simulink model "ground_sim"  (R2022a)
settings: Solver=FixedStepAuto  StartTime=0.0  StopTime=35  FixedStep=framePeriod_s  RelTol=1e-9
values from neighbouring files (symbols this model uses):
  framePeriod_s = 1/frameRate_hz    (= 0.02)    [autocode_setup.m]    (also in setup.m)
undefined symbols (not defined in the file or in its folder): accel_mps2, Aircraft, alt_msl_m, alt_wgs84_m, datetime, datevec, die_temp_c, Earth, Env, Fmu, gyro_radps, hdop, healthy, horz_acc_m, imu_healthy, InitCond, lat_rad, lon_rad, mag_healthy, mag_ut, ned_vel_mps, new_data, new_imu_data, new_mag_data, num_sats, pres_pa, spd_mps, Telem, tow_ms, track_acc_rad, track_rad, vdop, vel_acc_mps, vert_acc_m, week, WGS84
libraries: simulink x8, aerolibconvert2 x5, aerolibasang x3, aerolibtransform2 x2, aerolibgravity2 x2, aerolibatmos2 x1, sharedtransform x1, uavutilslib x1
(part 1 of 4)
settings Model: Creator=brian  LastModifiedBy=remoteuser
settings SolverCC: AlgebraicLoopSolver=TrustRegion
settings DataIOCC: SaveOutput=off  SignalLogging=off  DSMLogging=off  SaveTime=off  ReturnWorkspaceOutputsName=Data
settings OptimizationCC: DefaultParameterBehavior=Inlined  EnhancedBackFolding=on  PassReuseOutputArgsAs=Individual arguments  ZeroExternalMemoryAtStartup=off  ZeroInternalMemoryAtStartup=off  OptimizeBlockOrder=speed  DifferentSizesBufferReuse=on  OptimizationCustomize=off  EfficientTunableParamExpr=on
settings DebuggingCC: Int32ToFloatConvMsg=none  ParameterPrecisionLossMsg=none  ParameterTunabilityLossMsg=error  UnconnectedInputMsg=warning  UnconnectedOutputMsg=warning  UnconnectedLineMsg=warning  SFMachineParentedDataDiag=warning
settings SFSimCC: MATLABDynamicMemAlloc=off
settings RTWCC: SystemTargetFile=ert.tlc  GenCodeOnly=on  TemplateMakefile=ert_default_tmf  DLArmComputeVersion=19.05
settings CodeAppCC: ForceParamTrailComments=on  IgnoreCustomStorageClasses=off  OperatorAnnotations=on  SimulinkDataObjDesc=on  SFDataObjDesc=on  InsertBlockDesc=on
settings ERTTargetCC: TargetLangStandard=C99 (ISO)  GenerateSampleERTMain=on  InlinedParameterPlacement=NonHierarchical  ERTCustomFileTemplate=example_file_process.tlc

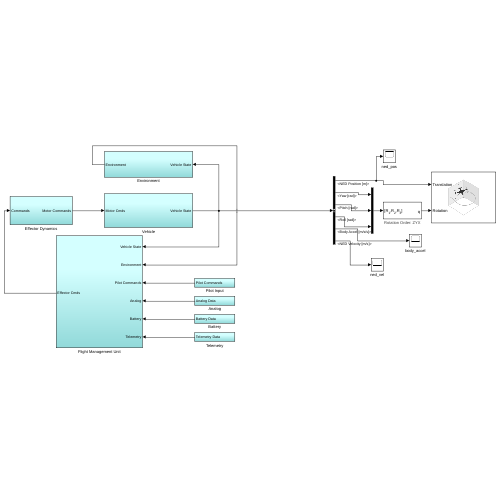
[thumbnail: Simulink's stored preview of the top-level diagram]
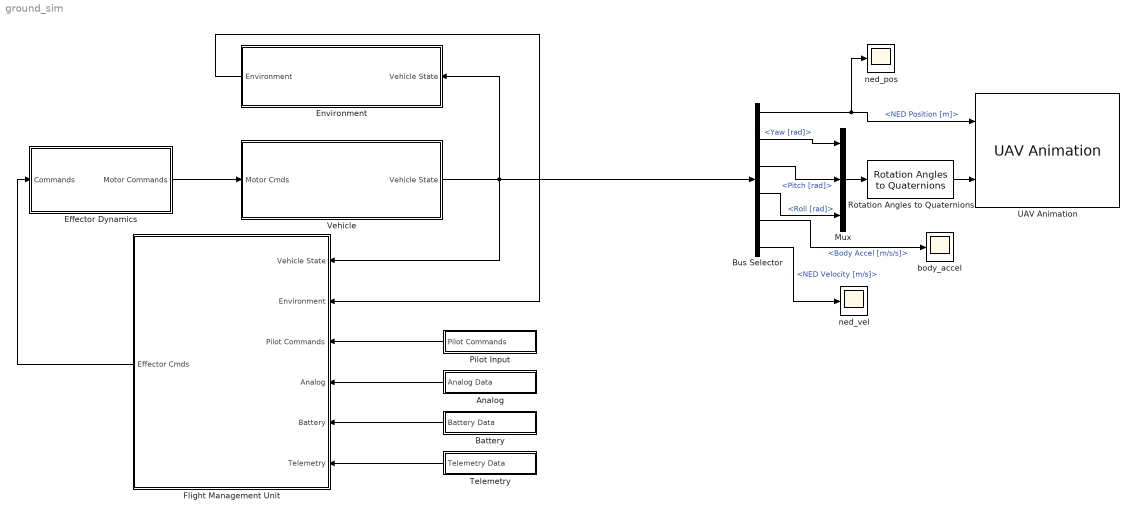
== system ground_sim ==
  Analog : Subsystem
  Battery : Subsystem
  Bus Selector : BusSelector  OutputSignals=NED Position [m],Yaw [rad],Pitch [rad],Roll [rad],Body Accel [m/s/s],NED Velocity [m/s]
  Effector Dynamics : Subsystem
  Environment : Subsystem
  Flight Management Unit : Subsystem
  Mux : Mux  Inputs=3
  Pilot Input : Subsystem
  Rotation Angles to Quaternions : sharedtransform/Rotation Angles to Quaternions  rotationOrder=ZYX  aMode=aMode
      settings: SourceProductBaseCode=AE,PW,DR,MT,VE
  Telemetry : Subsystem
  UAV Animation : uavutilslib/UAV Animation  UAVType=Multirotor  UAVSize=1  InertialZDirection=Down  SampleTime=-1
      settings: SourceProductBaseCode=UV
  Vehicle : Subsystem
  body_accel : Scope
  ned_pos : Scope
  ned_vel : Scope
  wires:
  Pilot Input/1(Pilot Commands) -> Flight Management Unit/3(Pilot Commands)
  Environment/1(Environment) -> Flight Management Unit/2(Environment)
  Effector Dynamics/1(Motor Commands) -> Vehicle/1(Motor Cmds)
  Telemetry/1(Telemetry Data) -> Flight Management Unit/6(Telemetry)
  Flight Management Unit/1(Effector Cmds) -> Effector Dynamics/1(Commands)
  Analog/1(Analog Data) -> Flight Management Unit/4(Analog)
  Battery/1(Battery Data) -> Flight Management Unit/5(Battery)
  Bus Selector/6 -> ned_vel/1  "<NED Velocity [m/s]>"
  Bus Selector/2 -> Mux/1  "<Yaw [rad]>"
  Bus Selector/5 -> body_accel/1  "<Body Accel [m/s/s]>"
  Rotation Angles to Quaternions/1 -> UAV Animation/2
  Bus Selector/3 -> Mux/2  "<Pitch [rad]>"
  Bus Selector/4 -> Mux/3  "<Roll [rad]>"
  Mux/1 -> Rotation Angles to Quaternions/1
  Bus Selector/1 -> ned_pos/1, UAV Animation/1  "<NED Position [m]>"
  Vehicle/1(Vehicle State) -> Bus Selector/1, Environment/1(Vehicle State), Flight Management Unit/1(Vehicle State)

== system ground_sim/Analog ==
  note: Raw voltages measured at the FMU, should be between
      | 0 and 3.3V
  Bus Creator : BusCreator  Inputs=1
  Constant : Constant  Value=zeros(1, Fmu.NUM_AIN)
  Mux : Mux  Inputs=2
  Random Number : RandomNumber  Mean=0.8  Variance=0.01  SampleTime=framePeriod_s
  Selector1 : Selector  InputPortWidth=Fmu.NUM_AIN  IndexOptions=Starting index (dialog)  Indices=[2]  OutputSizes=Fmu.NUM_AIN-1
  Analog Data : Outport
  wires:
  Bus Creator/1 -> Analog Data/1
  Mux/1 -> Bus Creator/1  "Voltages"
  Random Number/1 -> Mux/1
  Selector1/1 -> Mux/2
  Constant/1 -> Selector1/1  "Voltages"

== system ground_sim/Battery ==
  note: This is the amp draw from the battery
  note: The mRo Power Zero module
      | outputs 1V for 33.594 amps drawn
      | from the battery
  note: This is the voltage measured by the FMU
      | power port. It is typically the current, scaled
      | by the power module mA / volt
  note: This is the voltage
      | measured by the FMU at
      | the power port. It is typically
      | the battery voltage scaled by the
      | power module voltage divider.
  note: The mRo Power Zero module
      | outputs 1V for 15.30 V at the
      | battery
  Bus Creator : BusCreator  Inputs=2
  Constant : Constant  Value=Aircraft.Battery.voltage
  Constant1 : Constant  Value=42
  Constant2 : Constant
  Constant3 : Constant
  Divide : Product  Inputs=*/
  Divide1 : Product  Inputs=*/
  Battery Data : Outport
  wires:
  Bus Creator/1 -> Battery Data/1
  Constant2/1 -> Divide/2
  Constant1/1 -> Divide/1
  Divide/1 -> Bus Creator/2  "Current [V]"
  Divide1/1 -> Bus Creator/1  "Voltage [V]"
  Constant/1 -> Divide1/1
  Constant3/1 -> Divide1/2

== system ground_sim/Effector Dynamics ==
  Commands : Inport
  Bus Selector : BusSelector  OutputSignals=PWM.Cmds
  Selector1 : Selector  InputPortWidth=Aircraft.Eff.nPwm  IndexOptions=Index vector (dialog)  Indices=Aircraft.Motor.map  OutputSizes=1
  Motor Commands : Outport
  wires:
  Bus Selector/1 -> Selector1/1  "<Cmds>"
  Commands/1 -> Bus Selector/1
  Selector1/1 -> Motor Commands/1

== system ground_sim/Environment ==
  note: nT to uT conversion
  Vehicle State : Inport
  Angle Conversion4 : aerolibconvert2/Angle Conversion  IU=rad  OU=deg
  Angle Conversion5 : aerolibconvert2/Angle Conversion  IU=rad  OU=deg
  Bus Creator : BusCreator  Inputs=6
  Bus Selector : BusSelector  OutputSignals=Latitude [rad],Longitude [rad],Altitude WGS84 [m],Altitude MSL [m]
  COESA Atmosphere Model : aerolibatmos2/COESA Atmosphere Model  units=Metric (MKS)  spec=1976 COESA-extended U.S. Standard Atmosphere  model=Profile  profile_var=High temperature  profile_percent=1%  profile_alt=5 km (16404 ft)  envelope_var=High temperature  envelope_percent=1%  action=Warning
  Constant : Constant  Value=Env.wmm_nt
  Gain : Gain  Gain=1e-3
  Mux : Mux  Inputs=3
  "WGS84 Gravity Model  " : GravityWGS84
  Environment : Outport
  wires:
  [lon_deg] -> Mux/2
  COESA Atmosphere Model/4 -> Bus Creator/4  "Density [kg/m^3]"
  Mux/1 -> "WGS84 Gravity Model  "/1
  Bus Selector/3 -> [alt_wgs84_m]  "<Altitude WGS84 [m]>"
  Vehicle State/1 -> Bus Selector/1
  Bus Selector/2 -> Angle Conversion5/1  "<Longitude [rad]>"
  COESA Atmosphere Model/2 -> Bus Creator/2  "Speed of Sound [m/s]"
  Bus Selector/4 -> COESA Atmosphere Model/1  "<Altitude MSL [m]>"
  [alt_wgs84_m] -> Mux/3
  Angle Conversion4/1 -> [lat_deg]
  [lat_deg] -> Mux/1
  Bus Creator/1 -> Environment/1
  Constant/1 -> Gain/1
  Gain/1 -> Bus Creator/6  "Magnetic Field [uT]"
  "WGS84 Gravity Model  "/1 -> Bus Creator/5  "Gravity [m/s/s]"
  Bus Selector/1 -> Angle Conversion4/1  "<Latitude [rad]>"
  COESA Atmosphere Model/3 -> Bus Creator/3  "Pressure [Pa]"
  COESA Atmosphere Model/1 -> Bus Creator/1  "Temperature [K]"
  Angle Conversion5/1 -> [lon_deg]

== system ground_sim/Flight Management Unit ==
  Vehicle State : Inport
  Environment : Inport  Port=2
  Pilot Commands : Inport  Port=3
  Analog : Inport  Port=4
  Battery : Inport  Port=5
  Telemetry : Inport  Port=6
  Bus Selector1 : BusSelector  OutputSignals=Waypoint Reached
  Bus Selector2 : BusSelector  OutputSignals=Waypoint Reached,SBUS,PWM  OutputAsBus=on
  Navigation Filter Model : Subsystem
      settings: PortSchema="{\"entries\":[{\"content\":{\"sides\":[{\"content\":{\"connectorIds\":[]},\"type\":\"ConnectorPlacement.EquallySpacedRectSide\",\"uuid\":\"b20f7590-d69b-48b8-beb1-2fb7d3ab0357\"},{\"content\":{\"connectorIds\":[],\"side\":\"RIGHT\"},\"type\":\"ConnectorPlacement.EquallySpacedRectSide\",\"uuid\":\"07801f8a-7756-483e-a050-3c2fccc33404\"},{\"content\":{\"connectorIds\":[\"In1\",\"In2\"],\"side\":\"TOP\"},\"type\":\"ConnectorPlacement.EquallySpacedRectSide\",\"uuid\":\"ce3c3c94-ed36-4103-b079-69dcaeaf21e9\"},{\"content\":{\"connectorIds\":[\"Out1\"],\"side\":\"BOTTOM\"},\"type\":\"ConnectorPlacement.EquallySpacedRectSide\",\"uuid\":\"ba78b819-a471-4bc3-b479-e6a973cfe14f\"},{\"content\":{\"connectorIds\":[],\"side\":\"HIDDEN\"},\"type\":\"ConnectorPlacement.EquallySpacedRectSide\",\"uuid\":\"3cf915a5-25a1-4380-9090-9561533312da\"}]},\"type\":\"ConnectorPlacement.EquallySpacedConnector\",\"uuid\":\"7ef4ddaa-ccd2-4778-89ce-8b4685524e82\"}],\"packageUris\":[\"http://schema.mathworks.com/mf0/Connector/R2020b\"],\"version\":\"1.0\"}"
  Sensor Models : Subsystem
      settings: PortSchema="{\"entries\":[{\"content\":{\"sides\":[{\"content\":{\"connectorIds\":[]},\"type\":\"ConnectorPlacement.EquallySpacedRectSide\",\"uuid\":\"b20f7590-d69b-48b8-beb1-2fb7d3ab0357\"},{\"content\":{\"connectorIds\":[],\"side\":\"RIGHT\"},\"type\":\"ConnectorPlacement.EquallySpacedRectSide\",\"uuid\":\"07801f8a-7756-483e-a050-3c2fccc33404\"},{\"content\":{\"connectorIds\":[\"In1\",\"In2\",\"In3\",\"In4\",\"In5\"],\"side\":\"TOP\"},\"type\":\"ConnectorPlacement.EquallySpacedRectSide\",\"uuid\":\"ce3c3c94-ed36-4103-b079-69dcaeaf21e9\"},{\"content\":{\"connectorIds\":[\"Out1\"],\"side\":\"BOTTOM\"},\"type\":\"ConnectorPlacement.EquallySpacedRectSide\",\"uuid\":\"ba78b819-a471-4bc3-b479-e6a973cfe14f\"},{\"content\":{\"connectorIds\":[],\"side\":\"HIDDEN\"},\"type\":\"ConnectorPlacement.EquallySpacedRectSide\",\"uuid\":\"3cf915a5-25a1-4380-9090-9561533312da\"}]},\"type\":\"ConnectorPlacement.EquallySpacedConnector\",\"uuid\":\"7ef4ddaa-ccd2-4778-89ce-8b4685524e82\"}],\"packageUris\":[\"http://schema.mathworks.com/mf0/Connector/R2020b\"],\"version\":\"1.0\"}"
  Subsystem : Subsystem
  System Model : Subsystem
      settings: PortSchema="{\"entries\":[{\"content\":{\"sides\":[{\"content\":{\"connectorIds\":[]},\"type\":\"ConnectorPlacement.EquallySpacedRectSide\",\"uuid\":\"b20f7590-d69b-48b8-beb1-2fb7d3ab0357\"},{\"content\":{\"connectorIds\":[],\"side\":\"RIGHT\"},\"type\":\"ConnectorPlacement.EquallySpacedRectSide\",\"uuid\":\"07801f8a-7756-483e-a050-3c2fccc33404\"},{\"content\":{\"connectorIds\":[],\"side\":\"TOP\"},\"type\":\"ConnectorPlacement.EquallySpacedRectSide\",\"uuid\":\"ce3c3c94-ed36-4103-b079-69dcaeaf21e9\"},{\"content\":{\"connectorIds\":[\"Out1\"],\"side\":\"BOTTOM\"},\"type\":\"ConnectorPlacement.EquallySpacedRectSide\",\"uuid\":\"ba78b819-a471-4bc3-b479-e6a973cfe14f\"},{\"content\":{\"connectorIds\":[],\"side\":\"HIDDEN\"},\"type\":\"ConnectorPlacement.EquallySpacedRectSide\",\"uuid\":\"3cf915a5-25a1-4380-9090-9561533312da\"}]},\"type\":\"ConnectorPlacement.EquallySpacedConnector\",\"uuid\":\"7ef4ddaa-ccd2-4778-89ce-8b4685524e82\"}],\"packageUris\":[\"http://schema.mathworks.com/mf0/Connector/R2020b\"],\"version\":\"1.0\"}"
  Unit Delay : UnitDelay  SampleTime=-1  HasFrameUpgradeWarning=on
  Unit Delay1 : UnitDelay  SampleTime=-1  HasFrameUpgradeWarning=on
  Vehicle Management System (VMS) : Subsystem  TreatAsAtomicUnit=on
  Effector Cmds : Outport
  wires:
  Environment/1 -> Navigation Filter Model/1(Environment), Sensor Models/1(Environment)
  Vehicle State/1 -> Navigation Filter Model/2(Vehicle State), Sensor Models/2(Vehicle State)
  Sensor Models/1(Sensors) -> Unit Delay/1
  Navigation Filter Model/1(Navigation Filter Data) -> Unit Delay1/1
  System Model/1(System) -> Vehicle Management System (VMS)/1(System Data)
  Pilot Commands/1 -> Sensor Models/3(Inceptor Data)
  Telemetry/1 -> Subsystem/1(Bus)
  Vehicle Management System (VMS)/1(VMS Data) -> Bus Selector2/1
  Unit Delay/1 -> Vehicle Management System (VMS)/2(Sensor Data)
  Unit Delay1/1 -> Vehicle Management System (VMS)/3(Navigation Filter Data)
  Analog/1 -> Sensor Models/4(Analog Data)
  Battery/1 -> Sensor Models/5(Battery Data)
  Subsystem/1(Telemetry Data) -> Vehicle Management System (VMS)/4(Telemetry Data)
  Bus Selector1/1 -> Subsystem/2(<Waypoint Reached>)  "<Waypoint Reached>"
  Bus Selector2/1 -> Bus Selector1/1, Effector Cmds/1

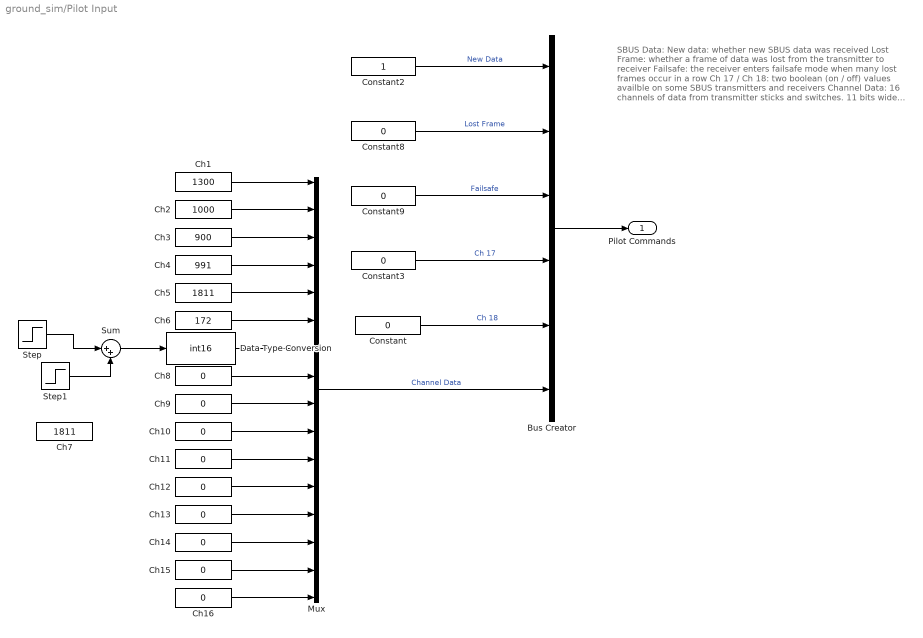
== system ground_sim/Pilot Input ==
  note: SBUS Data:
      | New data: whether new SBUS data was received
      | Lost Frame: whether a frame of data was lost from the transmitter to receiver
      | Failsafe: the receiver enters failsafe mode when many lost frames occur in a row
      | Ch 17 / Ch 18: two boolean (on / off) values availble on some SBUS transmitters and receivers
      | Channel Data: 16 channels of data from transmitter sticks and switches. 11 bits wide limiting values to 0 - 2048. Actual ranges may be different, for example, FrSky typically uses 172 - 1811 unless its range is extended to +/- 150%
  Bus Creator : BusCreator  Inputs=6
  Ch1 : Constant  Value=1300  OutDataTypeStr=int16  SampleTime=-1
  Ch{8..16} (9 alike) : Constant  Value=0  OutDataTypeStr=int16  SampleTime=-1
  Ch2 : Constant  Value=1000  OutDataTypeStr=int16  SampleTime=-1
  Ch3 : Constant  Value=900  OutDataTypeStr=int16  SampleTime=-1
  Ch4 : Constant  Value=991  OutDataTypeStr=int16  SampleTime=-1
  Ch5 : Constant  Value=1811  OutDataTypeStr=int16  SampleTime=-1
  Ch6 : Constant  Value=172  OutDataTypeStr=int16  SampleTime=-1
  Ch7 : Constant  Value=1811  OutDataTypeStr=int16  SampleTime=-1
  Constant : Constant  Value=0  OutDataTypeStr=int8
  Constant2 : Constant  OutDataTypeStr=boolean
  Constant3 : Constant  Value=0  OutDataTypeStr=boolean
  Constant8 : Constant  Value=0  OutDataTypeStr=boolean
  Constant9 : Constant  Value=0  OutDataTypeStr=boolean
  Data Type Conversion : DataTypeConversion  OutDataTypeStr=int16  SaturateOnIntegerOverflow=off  RndMeth=Floor
  Mux : Mux  Inputs=16
  Step : Step  Time=0  After=1811  SampleTime=0
  Step1 : Step  Time=2*framePeriod_s  After=-1811  SampleTime=0
  Sum : Sum  Inputs=|++
  Pilot Commands : Outport
  wires:
  Bus Creator/1 -> Pilot Commands/1
  Constant2/1 -> Bus Creator/1  "New Data"
  Constant8/1 -> Bus Creator/2  "Lost Frame"
  Constant9/1 -> Bus Creator/3  "Failsafe"
  Constant3/1 -> Bus Creator/4  "Ch 17"
  Constant/1 -> Bus Creator/5  "Ch 18"
  Mux/1 -> Bus Creator/6  "Channel Data"
  Ch1/1 -> Mux/1
  Ch16/1 -> Mux/16
  Ch15/1 -> Mux/15
  Ch14/1 -> Mux/14
  Ch13/1 -> Mux/13
  Ch12/1 -> Mux/12
  Ch11/1 -> Mux/11
  Ch10/1 -> Mux/10
  Ch9/1 -> Mux/9
  Ch8/1 -> Mux/8
  Data Type Conversion/1 -> Mux/7
  Ch6/1 -> Mux/6
  Ch4/1 -> Mux/4
  Ch2/1 -> Mux/2
  Ch3/1 -> Mux/3
  Ch5/1 -> Mux/5
  Step/1 -> Sum/1
  Step1/1 -> Sum/2
  Sum/1 -> Data Type Conversion/1

== system ground_sim/Telemetry ==
  Bus Creator : BusCreator  Inputs=11
  Constant1 : Constant  Value=0  OutDataTypeStr=boolean
  Constant10 : Constant  Value=Telem.Fence  OutDataTypeStr=Bus: MissionItem
  Constant11 : Constant  Value=Telem.Rally  OutDataTypeStr=Bus: MissionItem
  Constant2 : Constant  Value=0  OutDataTypeStr=boolean
  Constant3 : Constant  OutDataTypeStr=int16
  Constant4 : Constant  Value=0  OutDataTypeStr=int16
  Constant5 : Constant  Value=0  OutDataTypeStr=int16
  Constant6 : Constant  Value=0  OutDataTypeStr=int16
  Constant7 : Constant  Value=[0 0 0 0 0 0 0 0 0 0 1 1 1 0 0 0 0 0 0 0 0 0 0 0]  OutDataTypeStr=boolean
  Constant8 : Constant  Value=0  OutDataTypeStr=boolean
  Constant9 : Constant  Value=Telem.FlightPlan  OutDataTypeStr=Bus: MissionItem
  Telemetry Data : Outport
  wires:
  Bus Creator/1 -> Telemetry Data/1
  Constant8/1 -> Bus Creator/1  "Waypoints Updated"
  Constant1/1 -> Bus Creator/2  "Fence Updated"
  Constant2/1 -> Bus Creator/3  "Rally Points Updated"
  Constant3/1 -> Bus Creator/4  "Current Waypoint Index"
  Constant4/1 -> Bus Creator/5  "Number of Waypoints"
  Constant5/1 -> Bus Creator/6  "Number of Fence Points"
  Constant6/1 -> Bus Creator/7  "Number of Rally Points"
  Constant7/1 -> Bus Creator/8  "Parameters"
  Constant9/1 -> Bus Creator/9  "Flight Plan"
  Constant10/1 -> Bus Creator/10  "Fence"
  Constant11/1 -> Bus Creator/11  "Rally"

== system ground_sim/Vehicle ==
  note: The dynamics can be input here using the Motor Cmds as input
  Motor Cmds : Inport
  Bus Creator : BusCreator  Inputs=26
  Demux : Demux  Outputs=3
  Ground : Ground
  MATLAB Function : MATLAB Function  TreatAsAtomicUnit=on
  Vehicle Model : Subsystem
  Vehicle State : Outport
  wires:
  Vehicle Model/20(Angle of Attack Rate [rad/s]) -> Bus Creator/20  "Angle of Attack Rate [rad/s]"
  Vehicle Model/4(Altitude MSL [m]) -> Bus Creator/4  "Altitude MSL [m]"
  Vehicle Model/26(DCM_be) -> Bus Creator/26  "DCM_be"
  Vehicle Model/16(Dynamic Pressure [Pa]) -> Bus Creator/16  "Dynamic Pressure [Pa]"
  Vehicle Model/22(Sideslip Angle Rate [rad/s]) -> Bus Creator/22  "Sideslip Angle Rate [rad/s]"
  Vehicle Model/21(Sideslip Angle [rad]) -> Bus Creator/21  "Sideslip Angle [rad]"
  Vehicle Model/24(Flight Path Angle [rad]) -> Bus Creator/24  "Flight Path Angle [rad]"
  Vehicle Model/11(Yaw [rad]) -> MATLAB Function/2(phi), Bus Creator/11  "Yaw [rad]"
  Vehicle Model/18(Mach) -> Bus Creator/18  "Mach"
  Vehicle Model/5(Altitude AGL [m]) -> Bus Creator/5  "Altitude AGL [m]"
  Vehicle Model/6(NED Position [m]) -> Bus Creator/6  "NED Position [m]"
  Vehicle Model/23(Ground Track [rad]) -> Bus Creator/23  "Ground Track [rad]"
  Vehicle Model/10(Roll [rad]) -> Bus Creator/10  "Roll [rad]"
  Vehicle Model/7(NED Velocity [m/s]) -> Bus Creator/7  "NED Velocity [m/s]"
  Vehicle Model/17(Airspeed [m/s]) -> Bus Creator/17  "Airspeed [m/s]"
  Vehicle Model/15(Body Rotational Accel [rad/s/s]) -> Bus Creator/15  "Body Rotational Accel [rad/s/s]"
  Vehicle Model/14(Body Rotational Rate [rad/s]) -> Bus Creator/14  "Body Rotational Rate [rad/s]"
  Vehicle Model/13(Body Accel [m/s/s]) -> Bus Creator/13  "Body Accel [m/s/s]"
  Vehicle Model/9(Pitch [rad]) -> Bus Creator/9  "Pitch [rad]"
  Vehicle Model/8(NED Accel [m/s/s]) -> Bus Creator/8  "NED Accel [m/s/s]"
  Bus Creator/1 -> Vehicle State/1
  Vehicle Model/19(Angle of Attack [rad]) -> Bus Creator/19  "Angle of Attack [rad]"
  Vehicle Model/3(Altitude WGS84 [m]) -> Bus Creator/3  "Altitude WGS84 [m]"
  Motor Cmds/1 -> MATLAB Function/1(u)
  Vehicle Model/2(Longitude [rad]) -> Bus Creator/2  "Longitude [rad]"
  Vehicle Model/1(Latitude [rad]) -> Bus Creator/1  "Latitude [rad]"
  Vehicle Model/12(Body Velocity [m/s]) -> Bus Creator/12  "Body Velocity [m/s]"
  Vehicle Model/25(Ground Speed [m/s]) -> Bus Creator/25  "Ground Speed [m/s]"
  Demux/1 -> Vehicle Model/1(v_x [mps])
  Demux/2 -> Vehicle Model/2(v_y [mps])
  Demux/3 -> Vehicle Model/3(phi_dot [radps])
  Ground/1 -> Vehicle Model/5(Speed of Sound [m/s]), Vehicle Model/4(Density [kg/m^3])
  MATLAB Function/1(rate_out) -> Demux/1

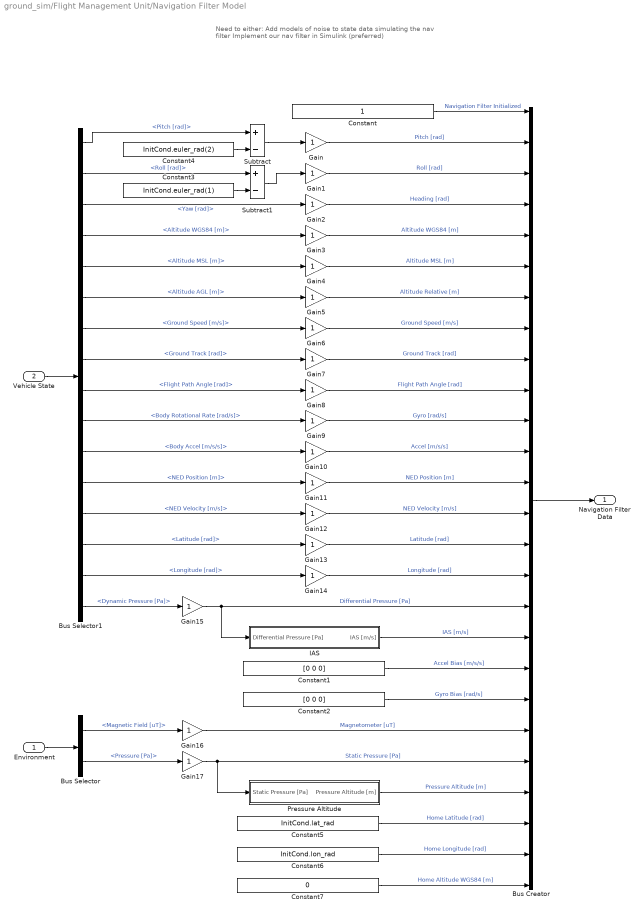
== system ground_sim/Flight Management Unit/Navigation Filter Model ==
  note: Need to either:
      | Add models of noise to state data simulating the nav filter
      | Implement our nav filter in Simulink (preferred)
  Environment : Inport
  Vehicle State : Inport  Port=2
  Bus Creator : BusCreator  Inputs=26
  Bus Selector : BusSelector  OutputSignals=Magnetic Field [uT],Pressure [Pa]
  Bus Selector1 : BusSelector  OutputSignals=Pitch [rad],Roll [rad],Yaw [rad],Altitude WGS84 [m],Altitude MSL [m],Altitude AGL [m],Ground Speed [m/s],Ground Track [rad],Flight Path Angle [rad],Body Rotational Rate [rad/s],Body Accel [m/s/s],NED Position [m],NED Velocity [m/s],Latitude [rad],Longitude [rad],Dynamic Pressure [Pa]
  Constant : Constant
  Constant1 : Constant  Value=[0 0 0]
  Constant2 : Constant  Value=[0 0 0]
  Constant3 : Constant  Value=InitCond.euler_rad(1)
  Constant4 : Constant  Value=InitCond.euler_rad(2)
  Constant5 : Constant  Value=InitCond.lat_rad
  Constant6 : Constant  Value=InitCond.lon_rad
  Constant7 : Constant  Value=0
  Gain{,1..17} (18 alike) : Gain
  IAS : Subsystem
  Pressure Altitude : Subsystem
  Subtract : Sum  Inputs=+-
  Subtract1 : Sum  Inputs=+-
  Navigation Filter Data : Outport
  wires:
  Environment/1 -> Bus Selector/1
  Bus Creator/1 -> Navigation Filter Data/1
  Vehicle State/1 -> Bus Selector1/1
  Constant/1 -> Bus Creator/1  "Navigation Filter Initialized"
  Bus Selector1/1 -> Subtract/1  "<Pitch [rad]>"
  Bus Selector1/2 -> Subtract1/1  "<Roll [rad]>"
  Bus Selector1/3 -> Gain2/1  "<Yaw [rad]>"
  Bus Selector1/4 -> Gain3/1  "<Altitude WGS84 [m]>"
  Bus Selector1/5 -> Gain4/1  "<Altitude MSL [m]>"
  Bus Selector1/6 -> Gain5/1  "<Altitude AGL [m]>"
  Bus Selector1/7 -> Gain6/1  "<Ground Speed [m/s]>"
  Bus Selector1/8 -> Gain7/1  "<Ground Track [rad]>"
  Bus Selector1/9 -> Gain8/1  "<Flight Path Angle [rad]>"
  Bus Selector1/10 -> Gain9/1  "<Body Rotational Rate [rad/s]>"
  Bus Selector1/11 -> Gain10/1  "<Body Accel [m/s/s]>"
  Bus Selector1/12 -> Gain11/1  "<NED Position [m]>"
  Bus Selector1/13 -> Gain12/1  "<NED Velocity [m/s]>"
  Bus Selector/2 -> Gain17/1  "<Pressure [Pa]>"
  Pressure Altitude/1(Pressure Altitude [m]) -> Bus Creator/23  "Pressure Altitude [m]"
  Bus Selector/1 -> Gain16/1  "<Magnetic Field [uT]>"
  Constant2/1 -> Bus Creator/20  "Gyro Bias [rad/s]"
  Constant1/1 -> Bus Creator/19  "Accel Bias [m/s/s]"
  IAS/1(IAS [m/s]) -> Bus Creator/18  "IAS [m/s]"
  Bus Selector1/16 -> Gain15/1  "<Dynamic Pressure [Pa]>"
  Bus Selector1/15 -> Gain14/1  "<Longitude [rad]>"
  Bus Selector1/14 -> Gain13/1  "<Latitude [rad]>"
  Gain/1 -> Bus Creator/2  "Pitch [rad]"
  Gain1/1 -> Bus Creator/3  "Roll [rad]"
  Gain2/1 -> Bus Creator/4  "Heading [rad]"
  Gain3/1 -> Bus Creator/5  "Altitude WGS84 [m]"
  Gain4/1 -> Bus Creator/6  "Altitude MSL [m]"
  Gain5/1 -> Bus Creator/7  "Altitude Relative [m]"
  Gain6/1 -> Bus Creator/8  "Ground Speed [m/s]"
  Gain7/1 -> Bus Creator/9  "Ground Track [rad]"
  Gain8/1 -> Bus Creator/10  "Flight Path Angle [rad]"
  Gain9/1 -> Bus Creator/11  "Gyro [rad/s]"
  Gain10/1 -> Bus Creator/12  "Accel [m/s/s]"
  Gain11/1 -> Bus Creator/13  "NED Position [m]"
  Gain12/1 -> Bus Creator/14  "NED Velocity [m/s]"
  Gain13/1 -> Bus Creator/15  "Latitude [rad]"
  Gain14/1 -> Bus Creator/16  "Longitude [rad]"
  Gain15/1 -> IAS/1(Differential Pressure [Pa]), Bus Creator/17  "Differential Pressure [Pa]"
  Gain16/1 -> Bus Creator/21  "Magnetometer [uT]"
  Gain17/1 -> Pressure Altitude/1(Static Pressure [Pa]), Bus Creator/22  "Static Pressure [Pa]"
  Subtract/1 -> Gain/1
  Subtract1/1 -> Gain1/1
  Constant3/1 -> Subtract1/2
  Constant4/1 -> Subtract/2
  Constant5/1 -> Bus Creator/24  "Home Latitude [rad]"
  Constant6/1 -> Bus Creator/25  "Home Longitude [rad]"
  Constant7/1 -> Bus Creator/26  "Home Altitude WGS84 [m]"

== system ground_sim/Flight Management Unit/Sensor Models ==
  Environment : Inport
  Vehicle State : Inport  Port=2
  Inceptor Data : Inport  Port=3
  Analog Data : Inport  Port=4
  Battery Data : Inport  Port=5
  Bus Creator : BusCreator  Inputs=8
  Bus Selector : BusSelector  OutputSignals=Body Rotational Rate [rad/s],Body Accel [m/s/s],DCM_be
  Bus Selector1 : BusSelector  OutputSignals=Latitude [rad],Longitude [rad],Altitude WGS84 [m],NED Velocity [m/s]
  Bus Selector2 : BusSelector  OutputSignals=Dynamic Pressure [Pa]
  Bus Selector3 : BusSelector  OutputSignals=Gravity [m/s/s],Magnetic Field [uT]
  Bus Selector4 : BusSelector  OutputSignals=Pressure [Pa]
  Constant : Constant  Value=Aircraft.Sensors.PitotStaticInstalled
  Diff Pressure Sensor : Subsystem
  GNSS : Subsystem
  IMU : Subsystem
  Static Pressure Sensor : Subsystem
  Sensors : Outport
  wires:
  Bus Creator/1 -> Sensors/1
  Vehicle State/1 -> Bus Selector2/1, Bus Selector1/1, Bus Selector/1
  Bus Selector/1 -> IMU/1(Body Rotational Rate [rad/s])  "<Body Rotational Rate [rad/s]>"
  Bus Selector/2 -> IMU/2(Body Accel [m/s/s])  "<Body Accel [m/s/s]>"
  Bus Selector/3 -> IMU/3(DCM_be)  "<DCM_be>"
  Bus Selector1/1 -> GNSS/1(Latitude [rad])  "<Latitude [rad]>"
  Bus Selector1/2 -> GNSS/2("Longitude [rad] ")  "<Longitude [rad]>"
  Bus Selector1/3 -> GNSS/3(Altitude WGS84 [m])  "<Altitude WGS84 [m]>"
  Bus Selector1/4 -> GNSS/4(NED Velocity [m/s])  "<NED Velocity [m/s]>"
  Bus Selector2/1 -> Diff Pressure Sensor/1(Pressure)  "<Dynamic Pressure [Pa]>"
  Environment/1 -> Bus Selector4/1, Bus Selector3/1
  Bus Selector3/1 -> IMU/4(Gravity [m/s/s])  "<Gravity [m/s/s]>"
  Bus Selector3/2 -> IMU/5(Magnetic Field [uT])  "<Magnetic Field [uT]>"
  Bus Selector4/1 -> Static Pressure Sensor/1(Pressure)  "<Pressure [Pa]>"
  IMU/1(IMU Data) -> Bus Creator/4  "IMU"
  GNSS/1(GNSS Data) -> Bus Creator/5  "GNSS"
  Inceptor Data/1 -> Bus Creator/2  "Inceptor"
  Diff Pressure Sensor/1(Pressure Data) -> Bus Creator/7  "Differential Pressure"
  Static Pressure Sensor/1(Pressure Data) -> Bus Creator/6  "Static Pressure"
  Constant/1 -> Bus Creator/1  "Pitot Static Installed"
  Analog Data/1 -> Bus Creator/3  "Analog"
  Battery Data/1 -> Bus Creator/8  "Battery"

== system ground_sim/Flight Management Unit/Subsystem ==
  Bus : Inport
  <Waypoint Reached> : Inport  Port=2
  Bus Creator : BusCreator  Inputs=11
  Bus Selector1 : BusSelector  OutputSignals=Waypoints Updated,Fence Updated,Rally Points Updated,Current Waypoint Index,Number of Waypoints,Number of Fence Points,Number of Rally Points,Parameters,Flight Plan,Fence,Rally
  Terminator : Terminator
  Triggered Subsystem : Subsystem  TreatAsAtomicUnit=on
  Unit Delay : UnitDelay  SampleTime=-1  HasFrameUpgradeWarning=on
  Unit Delay1 : UnitDelay  SampleTime=-1  HasFrameUpgradeWarning=on
  Telemetry Data : Outport
  wires:
  Bus Selector1/9 -> Bus Creator/9  "<Flight Plan>"
  Bus Selector1/3 -> Bus Creator/3  "<Rally Points Updated>"
  Bus Selector1/6 -> Bus Creator/6  "<Number of Fence Points>"
  <Waypoint Reached>/1 -> Unit Delay1/1
  Bus Selector1/11 -> Bus Creator/11  "<Rally>"
  Bus Selector1/10 -> Bus Creator/10  "<Fence>"
  Bus Selector1/4 -> Terminator/1  "<Current Waypoint Index>"
  Bus Selector1/8 -> Bus Creator/8  "<Parameters>"
  Bus Selector1/7 -> Bus Creator/7  "<Number of Rally Points>"
  Bus Selector1/2 -> Bus Creator/2  "<Fence Updated>"
  Bus Selector1/5 -> Bus Creator/5  "<Number of Waypoints>"
  Bus Selector1/1 -> Bus Creator/1  "<Waypoints Updated>"
  Triggered Subsystem/1(Wp++) -> Bus Creator/4, Unit Delay/1  "Current Waypoint Index"
  Bus/1 -> Bus Selector1/1
  Bus Creator/1 -> Telemetry Data/1
  Unit Delay/1 -> Triggered Subsystem/1(Wp)
  Unit Delay1/1 -> Triggered Subsystem/Trigger

== system ground_sim/Flight Management Unit/System Model ==
  Bus Creator : BusCreator  Inputs=8
  Clock : Clock
      settings: Decimation=1e6
  Constant : Constant  Value=5
  Constant1 : Constant  Value=5
  Constant2 : Constant  Value=5
  Constant3 : Constant  Value=Aircraft.Battery.voltage
  Constant4 : Constant  Value=framePeriod_s
  Gain : Gain  Gain=1e6
  Gain1 : Gain  Gain=1e6
  System : Outport
  wires:
  Clock/1 -> Bus Creator/8, Gain/1  "System Time [s]"
  Bus Creator/1 -> System/1
  Constant4/1 -> Bus Creator/2, Gain1/1  "Frame Time [s]"
  Gain1/1 -> Bus Creator/1  "Frame Time [us]"
  Constant3/1 -> Bus Creator/3  "Input Voltage"
  Constant2/1 -> Bus Creator/4  "Regulated Voltage"
  Constant1/1 -> Bus Creator/5  "PWM Voltage"
  Constant/1 -> Bus Creator/6  "SBUS Voltage"
  Gain/1 -> Bus Creator/7  "System Time [us]"

== system ground_sim/Flight Management Unit/Vehicle Management System (VMS) ==
  System Data : Inport
  Sensor Data : Inport  Port=2
  Navigation Filter Data : Inport  Port=3
  Telemetry Data : Inport  Port=4
  Variant Subsystem : Subsystem  Variant=on
  VMS Data : Outport
  wires:
  Variant Subsystem/1(VMS Data) -> VMS Data/1
  System Data/1 -> Variant Subsystem/1(System Data)
  Sensor Data/1 -> Variant Subsystem/2(Sensor Data)
  Navigation Filter Data/1 -> Variant Subsystem/3(Navigation Filter Data)
  Telemetry Data/1 -> Variant Subsystem/4(Telemetry Data)

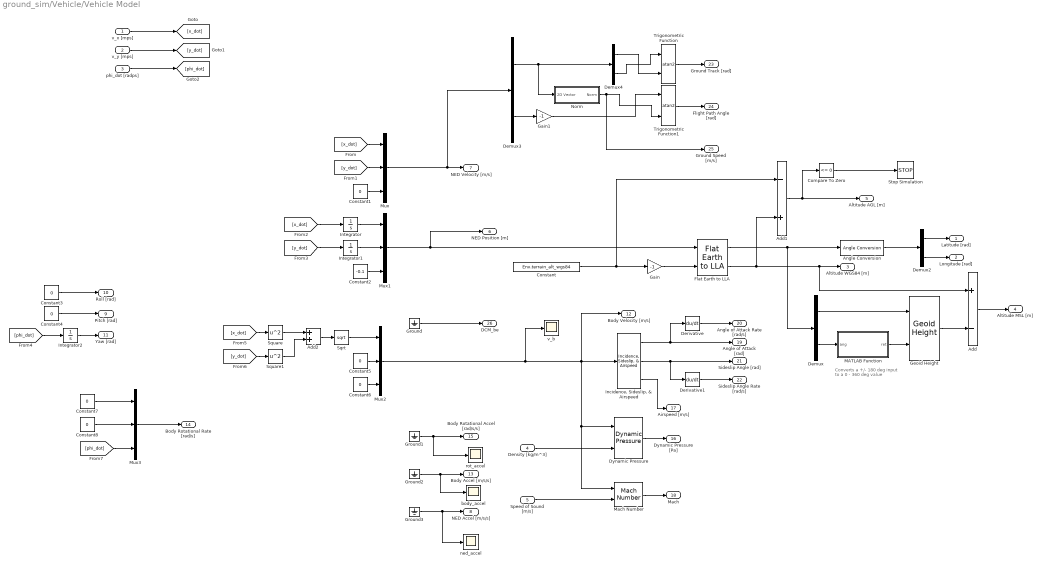
== system ground_sim/Vehicle/Vehicle Model ==
  note: Converts a +/- 180 deg
      | input to a 0 - 360 deg value
  v_x [mps] : Inport
  v_y [mps] : Inport  Port=2
  phi_dot [radps] : Inport  Port=3
  Density [kg/m^3] : Inport  Port=4
  Speed of Sound [m/s] : Inport  Port=5
  Add : Sum  Inputs=+-
  Add1 : Sum  Inputs=-+
  Add2 : Sum
  Angle Conversion : aerolibconvert2/Angle Conversion  IU=deg  OU=rad
  Compare To Zero : simulink/Logic and Bit Operations/Compare To Zero  relop=<=  OutDataTypeStr=boolean
  Constant : Constant  Value=Env.terrain_alt_wgs84
  Constant{1,3..8} (7 alike) : Constant  Value=0
  Constant2 : Constant  Value=-0.1
  Demux : Demux  Outputs=2
  Demux2 : Demux  Outputs=2
  Demux3 : Demux  Outputs=[2 1]
  Demux4 : Demux  Outputs=2
  Derivative : Derivative
  Derivative1 : Derivative
  Dynamic Pressure : aerolibasang/Dynamic Pressure
  Flat Earth to LLA : aerolibtransform2/Flat Earth to LLA  units=Metric (MKS)  ptype=Earth (WGS84)  F=1/298.257223563  R=6378137  refPosPort=off  LL0=[rad2deg(InitCond.lat_rad) rad2deg(InitCond.lon_rad)]  psi=0
  Gain : Gain  Gain=-1
  Gain1 : Gain  Gain=-1
  Geoid Height : aerolibgravity2/Geoid Height  units=Metric (MKS)  gtype=EGM2008  datafile='geoidegm96grid'  dtype=double  action=Warning
      settings: SourceProductBaseCode=AE
  Ground{,1..3} (4 alike) : Ground
  "Incidence, Sideslip, & Airspeed" : aerolibasang/Incidence, Sideslip, & Airspeed
  Integrator : Integrator
  Integrator1 : Integrator
  Integrator2 : Integrator
  MATLAB Function : MATLAB Function  TreatAsAtomicUnit=on
  Mach Number : aerolibasang/Mach Number
      settings: SourceProductBaseCode=AE
  Mux{,1..3} (4 alike) : Mux  Inputs=3
  Norm : Subsystem
  Sqrt : Sqrt
  Square : Math  Operator=square
  Square1 : Math  Operator=square
  Stop Simulation : Stop
  Trigonometric Function : Trigonometry  Operator=atan2
  Trigonometric Function1 : Trigonometry  Operator=atan2
  body_accel : Scope
  ned_accel : Scope
  rot_accel : Scope
  v_b : Scope
  Latitude [rad] : Outport
  Longitude [rad] : Outport  Port=2
  Altitude WGS84 [m] : Outport  Port=3
  Altitude MSL [m] : Outport  Port=4
  Altitude AGL [m] : Outport  Port=5
  NED Position [m] : Outport  Port=6
  NED Velocity [m/s] : Outport  Port=7
  NED Accel [m/s/s] : Outport  Port=8
  Pitch [rad] : Outport  Port=9
  Roll [rad] : Outport  Port=10
  Yaw [rad] : Outport  Port=11
  Body Velocity [m/s] : Outport  Port=12
  Body Accel [m/s/s] : Outport  Port=13
  Body Rotational Rate [rad/s] : Outport  Port=14
  Body Rotational Accel [rad/s/s] : Outport  Port=15
  Dynamic Pressure [Pa] : Outport  Port=16
  Airspeed [m/s] : Outport  Port=17
  Mach : Outport  Port=18
  Angle of Attack [rad] : Outport  Port=19
  Angle of Attack Rate [rad/s] : Outport  Port=20
  Sideslip Angle [rad] : Outport  Port=21
  Sideslip Angle Rate [rad/s] : Outport  Port=22
  Ground Track [rad] : Outport  Port=23
  Flight Path Angle [rad] : Outport  Port=24
  Ground Speed [m/s] : Outport  Port=25
  DCM_be : Outport  Port=26
  wires:
  v_x [mps]/1 -> [x_dot]
  phi_dot [radps]/1 -> [phi_dot]
  Mux2/1 -> v_b/1, Body Velocity [m/s]/1, "Incidence, Sideslip, & Airspeed"/1, Dynamic Pressure/1, Mach Number/1
  Flat Earth to LLA/1 -> Demux/1, Angle Conversion/1
  Flat Earth to LLA/2 -> Add1/2, Add/1, Altitude WGS84 [m]/1
  Geoid Height/1 -> Add/2
  Demux/2 -> MATLAB Function/1(ang)
  Demux/1 -> Geoid Height/1
  "Incidence, Sideslip, & Airspeed"/3 -> Airspeed [m/s]/1
  Density [kg/m^3]/1 -> Dynamic Pressure/2
  Angle Conversion/1 -> Demux2/1
  Ground/1 -> DCM_be/1
  Constant3/1 -> Roll [rad]/1
  Constant4/1 -> Pitch [rad]/1
  Integrator2/1 -> Yaw [rad]/1
  Dynamic Pressure/1 -> Dynamic Pressure [Pa]/1
  "Incidence, Sideslip, & Airspeed"/1 -> Derivative/1, Angle of Attack [rad]/1
  "Incidence, Sideslip, & Airspeed"/2 -> Derivative1/1, Sideslip Angle [rad]/1
  Add/1 -> Altitude MSL [m]/1
  Gain/1 -> Flat Earth to LLA/2
  Demux2/2 -> Longitude [rad]/1
  Demux2/1 -> Latitude [rad]/1
  Mux1/1 -> NED Position [m]/1, Flat Earth to LLA/1
  Mux3/1 -> Body Rotational Rate [rad/s]/1
  Ground1/1 -> rot_accel/1, Body Rotational Accel [rad/s/s]/1
  Mux/1 -> NED Velocity [m/s]/1, Demux3/1
  MATLAB Function/1(ret) -> Geoid Height/2
  Demux3/1 -> Norm/1(2D Vector), Demux4/1
  Trigonometric Function/1 -> Ground Track [rad]/1
  Demux3/2 -> Gain1/1
  Gain1/1 -> Trigonometric Function1/1
  Norm/1(Norm) -> Ground Speed [m/s]/1, Trigonometric Function1/2
  Trigonometric Function1/1 -> Flight Path Angle [rad]/1
  Ground3/1 -> ned_accel/1, NED Accel [m/s/s]/1
  Speed of Sound [m/s]/1 -> Mach Number/2
  Mach Number/1 -> Mach/1
  Derivative/1 -> Angle of Attack Rate [rad/s]/1
  Derivative1/1 -> Sideslip Angle Rate [rad/s]/1
  Constant/1 -> Add1/1, Gain/1
  Add1/1 -> Compare To Zero/1, Altitude AGL [m]/1
  Compare To Zero/1 -> Stop Simulation/1
  Demux4/1 -> Trigonometric Function/2
  Demux4/2 -> Trigonometric Function/1
  Ground2/1 -> body_accel/1, Body Accel [m/s/s]/1
  Constant1/1 -> Mux/3
  [x_dot] -> Mux/1
  v_y [mps]/1 -> [y_dot]
  [y_dot] -> Mux/2
  Constant2/1 -> Mux1/3
  Integrator/1 -> Mux1/1
  [x_dot] -> Integrator/1
  Integrator1/1 -> Mux1/2
  [y_dot] -> Integrator1/1
  [phi_dot] -> Integrator2/1
  Constant5/1 -> Mux2/2
  Constant6/1 -> Mux2/3
  [x_dot] -> Square/1
  [y_dot] -> Square1/1
  Square/1 -> Add2/1
  Square1/1 -> Add2/2
  Add2/1 -> Sqrt/1
  Sqrt/1 -> Mux2/1
  Constant8/1 -> Mux3/2
  Constant7/1 -> Mux3/1
  [phi_dot] -> Mux3/3

== system ground_sim/Flight Management Unit/Navigation Filter Model/IAS ==
  note: Avoid negative values
  Differential Pressure [Pa] : Inport
  Add : Sum
  Constant : Constant  OutDataTypeStr=double
  Constant1 : Constant  Value=2/7  OutDataTypeStr=double
  Constant2 : Constant  OutDataTypeStr=double
  Divide : Product  Inputs=*/
  Multiply : Gain  Gain=5
  Pow : Math  Operator=pow  RndMeth=Zero
  Product : Product
  Saturation : Saturate  UpperLimit=inf  LowerLimit=0
  Sqrt : Sqrt
  Standard Sea Level Pressure [Pa] : Constant  Value=101325  OutDataTypeStr=double
  Standard Sea Level Speed of Sound [m/s] : Constant  Value=340.29  OutDataTypeStr=double
  Subtract : Sum  Inputs=+-
  IAS [m/s] : Outport
  wires:
  Differential Pressure [Pa]/1 -> Saturation/1
  Saturation/1 -> Divide/1
  Standard Sea Level Pressure [Pa]/1 -> Divide/2
  Divide/1 -> Add/1
  Constant/1 -> Add/2
  Constant1/1 -> Pow/2
  Add/1 -> Pow/1
  Pow/1 -> Subtract/1
  Constant2/1 -> Subtract/2
  Subtract/1 -> Multiply/1
  Multiply/1 -> Sqrt/1
  Sqrt/1 -> Product/1
  Product/1 -> IAS [m/s]/1
  Standard Sea Level Speed of Sound [m/s]/1 -> Product/2

== system ground_sim/Flight Management Unit/Navigation Filter Model/Pressure Altitude ==
  note: Avoid negative values
  Static Pressure [Pa] : Inport
  Acceleration due to Gravity [m/s/s] : Constant  Value=9.80665  OutDataTypeStr=double
  Constant : Constant  OutDataTypeStr=double
  Divide : Product  Inputs=*/
  Divide1 : Product  Inputs=*/
  Divide2 : Product  Inputs=*/*
  Gas Constant [J/kg/mol] : Constant  Value=8.31446261815324  OutDataTypeStr=double
  Lapse Rate [K/m] : Constant  Value=0.0065  OutDataTypeStr=double
  Lapse Rate [K/m]1 : Constant  Value=0.0065  OutDataTypeStr=double
  Molecular Mass Air [kg/mol] : Constant  Value=0.0289644  OutDataTypeStr=double
  Pow : Math  Operator=pow  RndMeth=Zero
  Product : Product
  Product1 : Product
  Saturation1 : Saturate  UpperLimit=inf  LowerLimit=0
  Standard Sea Level Pressure [Pa] : Constant  Value=101325  OutDataTypeStr=double
  Standard Sea Level Temperature [K] : Constant  Value=288.15  OutDataTypeStr=double
  Subtract : Sum  Inputs=+-
  Pressure Altitude [m] : Outport
  wires:
  Static Pressure [Pa]/1 -> Saturation1/1
  Saturation1/1 -> Divide/1
  Standard Sea Level Pressure [Pa]/1 -> Divide/2
  Divide/1 -> Pow/1
  Product1/1 -> Divide1/1
  Product/1 -> Divide1/2
  Molecular Mass Air [kg/mol]/1 -> Product/1
  Acceleration due to Gravity [m/s/s]/1 -> Product/2
  Gas Constant [J/kg/mol]/1 -> Product1/2
  Lapse Rate [K/m]/1 -> Product1/1
  Divide1/1 -> Pow/2
  Pow/1 -> Subtract/2
  Constant/1 -> Subtract/1
  Subtract/1 -> Divide2/3
  Divide2/1 -> Pressure Altitude [m]/1
  Lapse Rate [K/m]1/1 -> Divide2/2
  Standard Sea Level Temperature [K]/1 -> Divide2/1

== system ground_sim/Flight Management Unit/Sensor Models/Diff Pressure Sensor ==
  Pressure : Inport
  Add : Sum  Inputs=+++
  Band-Limited White Noise : simulink/Sources/Band-Limited White Noise  Cov=Aircraft.Sensors.DiffPres.noise_pa  Ts=0.1  seed=[23341]
  Bus Creator : BusCreator  Inputs=4
  Bus Creator1 : BusCreator  Inputs=4
  Constant : Constant  Value=Aircraft.Sensors.DiffPres.bias_pa
  Constant1 : Constant  Value=Aircraft.Sensors.DiffPres.scale_factor
  Constant2 : Constant  Value=23
  Constant3 : Constant
  Constant4 : Constant
  Constant{5..8} (4 alike) : Constant  Value=0
  Constant9 : Constant  Value=Aircraft.Sensors.PitotStaticInstalled
  Product : Product
  Saturation : Saturate  UpperLimit=Aircraft.Sensors.DiffPres.upper_limit_pa  LowerLimit=Aircraft.Sensors.DiffPres.lower_limit_pa
  Switch : Switch  Criteria=u2 > Threshold  SaturateOnIntegerOverflow=off  InputSameDT=off
  Pressure Data : Outport
  wires:
  Switch/1 -> Pressure Data/1
  Constant9/1 -> Switch/2
  Bus Creator/1 -> Switch/1
  Bus Creator1/1 -> Switch/3
  Constant7/1 -> Bus Creator1/1  "New Data"
  Constant6/1 -> Bus Creator1/2  "Healthy"
  Constant5/1 -> Bus Creator1/4  "Die Temperature [C]"
  Constant8/1 -> Bus Creator1/3  "Pressure [Pa]"
  Constant1/1 -> Product/2
  Pressure/1 -> Product/1
  Product/1 -> Add/3
  Add/1 -> Saturation/1
  Constant/1 -> Add/2
  Band-Limited White Noise/1 -> Add/1
  Saturation/1 -> Bus Creator/3  "Pressure [Pa]"
  Constant2/1 -> Bus Creator/4  "Die Temperature [C]"
  Constant3/1 -> Bus Creator/2  "Healthy"
  Constant4/1 -> Bus Creator/1  "New Data"

== system ground_sim/Flight Management Unit/Sensor Models/GNSS ==
  note: Simulates the lower sampling rate of GNSS receivers
  Latitude [rad] : Inport
  "Longitude [rad] " : Inport  Port=2
  Altitude WGS84 [m] : Inport  Port=3
  NED Velocity [m/s] : Inport  Port=4
  Band-Limited White Noise : simulink/Sources/Band-Limited White Noise  Cov=[Aircraft.Sensors.Gnss.horz_accuracy_m Aircraft.Sensors.Gnss.horz_accuracy_m Aircraft.Sensors.Gnss.vert_accuracy_m]  Ts=0.1  seed=[23341]
  Band-Limited White Noise2 : simulink/Sources/Band-Limited White Noise  Cov=Aircraft.Sensors.Gnss.vel_accuracy_mps * ones(3, 1)  Ts=0.1  seed=[23341]
  Bus Creator : BusCreator  Inputs=19
  Clock : Clock
  Pulse Generator : DiscretePulseGenerator  PulseType=Time based  Period=1/Aircraft.Sensors.Gnss.sample_rate_hz  PulseWidth=5
  Triggered Subsystem : Subsystem  TreatAsAtomicUnit=on
  GNSS Data : Outport
  wires:
  Bus Creator/1 -> GNSS Data/1
  NED Velocity [m/s]/1 -> Triggered Subsystem/4(NED Velocity [m/s])
  Altitude WGS84 [m]/1 -> Triggered Subsystem/3(Altitude WGS84 [m])
  "Longitude [rad] "/1 -> Triggered Subsystem/2("Longitude [rad] ")
  Clock/1 -> Triggered Subsystem/7(clock)
  Band-Limited White Noise/1 -> Triggered Subsystem/5(Position Noise [m])
  Pulse Generator/1 -> Triggered Subsystem/Trigger
  Band-Limited White Noise2/1 -> Triggered Subsystem/6(Velocity Noise [m/s])
  Latitude [rad]/1 -> Triggered Subsystem/1(Latitude [rad])
  Triggered Subsystem/1(New Data) -> Bus Creator/1  "New Data"
  Triggered Subsystem/2(Healthy) -> Bus Creator/2  "Healthy"
  Triggered Subsystem/3(Fix) -> Bus Creator/3  "Fix"
  Triggered Subsystem/4(Num Satellites) -> Bus Creator/4  "Num Satellites"
  Triggered Subsystem/5(Week) -> Bus Creator/5  "Week"
  Triggered Subsystem/6(TOW [ms]) -> Bus Creator/6  "TOW [ms]"
  Triggered Subsystem/7(Alt WGS84 [m]) -> Bus Creator/7  "Altitude WGS84 [m]"
  Triggered Subsystem/8(Alt MSL [m]) -> Bus Creator/8  "Altitude MSL [m]"
  Triggered Subsystem/9(HDOP) -> Bus Creator/9  "HDOP"
  Triggered Subsystem/10(VDOP) -> Bus Creator/10  "VDOP"
  Triggered Subsystem/11(Track [rad]) -> Bus Creator/11  "Track [rad]"
  Triggered Subsystem/12(Speed [m/s]) -> Bus Creator/12  "Speed [m/s]"
  Triggered Subsystem/13(Horizontal Accuracy [m]) -> Bus Creator/13  "Horizontal Accuracy [m]"
  Triggered Subsystem/14(Vertical Accuracy [m]) -> Bus Creator/14  "Vertical Accuracy [m]"
  Triggered Subsystem/15(Velocity Accuracy [m/s]) -> Bus Creator/15  "Velocity Accuracy [m/s]"
  Triggered Subsystem/16(Track Accuracy [rad]) -> Bus Creator/16  "Track Accuracy [rad]"
  Triggered Subsystem/17(NED Vel [m/s]) -> Bus Creator/17  "NED Velocity [m/s]"
  Triggered Subsystem/18(Lat [rad]) -> Bus Creator/18  "Latitude [rad]"
  Triggered Subsystem/19(Lon [rad]) -> Bus Creator/19  "Longitude [rad]"

== system ground_sim/Flight Management Unit/Sensor Models/IMU ==
  Body Rotational Rate [rad/s] : Inport
  Body Accel [m/s/s] : Inport  Port=2
  DCM_be : Inport  Port=3
  Gravity [m/s/s] : Inport  Port=4
  Magnetic Field [uT] : Inport  Port=5
  Accelerometer : Subsystem
  Bus Creator : BusCreator  Inputs=8
  Constant{,1..3} (4 alike) : Constant
  Constant4 : Constant  Value=23
  Gyro : Subsystem
  Magnetometer : Subsystem
  Product1 : Product  Multiplication=Matrix(*)
  Product2 : Product  Multiplication=Matrix(*)
  Reshape : Reshape  OutputDimensionality=Column vector (2-D)
  Reshape1 : Reshape
  Reshape2 : Reshape
  Reshape3 : Reshape  OutputDimensionality=Column vector (2-D)
  IMU Data : Outport
  wires:
  Body Accel [m/s/s]/1 -> Accelerometer/1(Body Accel [m/s/s]), Gyro/2(Body Accel [m/s/s])
  DCM_be/1 -> Product2/1, Product1/1
  Gravity [m/s/s]/1 -> Reshape/1
  Bus Creator/1 -> IMU Data/1
  Product2/1 -> Reshape1/1
  Reshape1/1 -> Accelerometer/2(Gravitational Accel in Body Frame [m/s/s])
  Body Rotational Rate [rad/s]/1 -> Gyro/1(Body Rotational Rate [rad/s])
  Reshape2/1 -> Magnetometer/1(Body Magnetic Field [uT])
  Product1/1 -> Reshape2/1
  Reshape3/1 -> Product1/2
  Magnetic Field [uT]/1 -> Reshape3/1
  Magnetometer/1(Magnetometer [uT]) -> Bus Creator/8  "Magnetometer [uT]"
  Accelerometer/1(Accelerometer [m/s/s]) -> Bus Creator/7  "Accelerometer [m/s/s]"
  Gyro/1(Gyro [rad/s]) -> Bus Creator/6  "Gyro [rad/s]"
  Reshape/1 -> Product2/2
  Constant1/1 -> Bus Creator/2  "New Magnetometer Data"
  Constant/1 -> Bus Creator/1  "New IMU Data"
  Constant2/1 -> Bus Creator/3  "IMU Healthy"
  Constant3/1 -> Bus Creator/4  "Magnetometer Healthy"
  Constant4/1 -> Bus Creator/5  "Die Temperature [C]"

== system ground_sim/Flight Management Unit/Sensor Models/Static Pressure Sensor ==
  Pressure : Inport
  Add : Sum  Inputs=+++
  Band-Limited White Noise : simulink/Sources/Band-Limited White Noise  Cov=Aircraft.Sensors.StaticPres.noise_pa  Ts=0.1  seed=[23341]
  Bus Creator : BusCreator  Inputs=4
  Constant : Constant  Value=Aircraft.Sensors.StaticPres.bias_pa
  Constant1 : Constant  Value=Aircraft.Sensors.StaticPres.scale_factor
  Constant2 : Constant  Value=23
  Constant3 : Constant
  Constant4 : Constant
  Product : Product
  Saturation : Saturate  UpperLimit=Aircraft.Sensors.StaticPres.upper_limit_pa  LowerLimit=Aircraft.Sensors.StaticPres.lower_limit_pa
  Pressure Data : Outport
  wires:
  Constant4/1 -> Bus Creator/1  "New Data"
  Constant3/1 -> Bus Creator/2  "Healthy"
  Constant2/1 -> Bus Creator/4  "Die Temperature [C]"
  Saturation/1 -> Bus Creator/3  "Pressure [Pa]"
  Band-Limited White Noise/1 -> Add/1
  Constant/1 -> Add/2
  Add/1 -> Saturation/1
  Product/1 -> Add/3
  Pressure/1 -> Product/1
  Constant1/1 -> Product/2
  Bus Creator/1 -> Pressure Data/1

== system ground_sim/Flight Management Unit/Subsystem/Triggered Subsystem ==
  Wp : Inport
  Trigger : TriggerPort  VariantControl=(inherit)
  Constant : Constant  OutDataTypeStr=int16
  Sum : Sum  Inputs=|++  AccumDataTypeStr=uint16
  Wp++ : Outport
  wires:
  Wp/1 -> Sum/1
  Constant/1 -> Sum/2
  Sum/1 -> Wp++/1

== system ground_sim/Flight Management Unit/Vehicle Management System (VMS)/Variant Subsystem ==
  System Data : Inport
  Sensor Data : Inport  Port=2
  Navigation Filter Data : Inport  Port=3
  Telemetry Data : Inport  Port=4
  FMU v1 : Subsystem  VariantControl=Fmu.version == 1
  FMU v2 : Subsystem  VariantControl=Fmu.version == 3
  FMU v2 Beta : Subsystem  VariantControl=Fmu.version == 2
  VMS Data : Outport

== system ground_sim/Vehicle/Vehicle Model/Norm ==
  2D Vector : Inport
  Product : Product
  Sqrt : Sqrt
  Sum of Elements : Sum  Inputs=+
  Norm : Outport
  wires:
  2D Vector/1 -> Product/2, Product/1
  Product/1 -> Sum of Elements/1
  Sum of Elements/1 -> Sqrt/1
  Sqrt/1 -> Norm/1

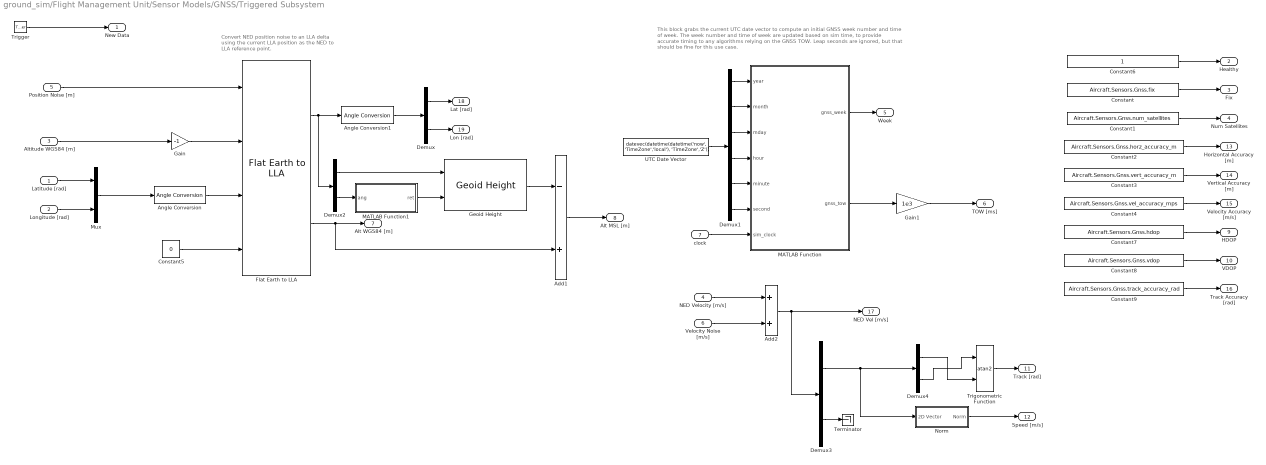
== system ground_sim/Flight Management Unit/Sensor Models/GNSS/Triggered Subsystem ==
  note: This block grabs the current UTC date vector to compute an initial GNSS week number
      | and time of week. The week number and time of week are updated based on sim time, to provide accurate timing to any algorithms relying on the GNSS TOW. Leap seconds are ignored, but that should be fine for this use case.
  note: Convert NED position noise to an LLA delta
      | using the current LLA position as the NED to
      | LLA reference point.
  Latitude [rad] : Inport
  "Longitude [rad] " : Inport  Port=2
  Altitude WGS84 [m] : Inport  Port=3
  NED Velocity [m/s] : Inport  Port=4  PortDimensions=3
  Position Noise [m] : Inport  Port=5  PortDimensions=3
  Velocity Noise [m/s] : Inport  Port=6  PortDimensions=3
  clock : Inport  Port=7
  Trigger : TriggerPort  VariantControl=Variant  ShowOutputPort=on
  Add1 : Sum  Inputs=-+
  Add2 : Sum
  Angle Conversion : aerolibconvert2/Angle Conversion  IU=rad  OU=deg
  Angle Conversion1 : aerolibconvert2/Angle Conversion  IU=deg  OU=rad
  Constant : Constant  Value=Aircraft.Sensors.Gnss.fix
  Constant1 : Constant  Value=Aircraft.Sensors.Gnss.num_satellites
  Constant2 : Constant  Value=Aircraft.Sensors.Gnss.horz_accuracy_m
  Constant3 : Constant  Value=Aircraft.Sensors.Gnss.vert_accuracy_m
  Constant4 : Constant  Value=Aircraft.Sensors.Gnss.vel_accuracy_mps
  Constant5 : Constant  Value=0
  Constant6 : Constant
  Constant7 : Constant  Value=Aircraft.Sensors.Gnss.hdop
  Constant8 : Constant  Value=Aircraft.Sensors.Gnss.vdop
  Constant9 : Constant  Value=Aircraft.Sensors.Gnss.track_accuracy_rad
  Demux : Demux  Outputs=2
  Demux1 : Demux  Outputs=6
  Demux2 : Demux  Outputs=2
  Demux3 : Demux  Outputs=[2 1]
  Demux4 : Demux  Outputs=2
  Flat Earth to LLA : aerolibtransform2/Flat Earth to LLA  units=Metric (MKS)  ptype=Earth (WGS84)  F=1/298.257223563  R=6378137  refPosPort=on  LL0=[0 10]  psi=0
  Gain : Gain  Gain=-1
  Gain1 : Gain  Gain=1e3
  Geoid Height : aerolibgravity2/Geoid Height  units=Metric (MKS)  gtype=EGM96  datafile='geoidegm96grid'  dtype=double  action=Warning
      settings: SourceProductBaseCode=AE
  MATLAB Function : MATLAB Function  TreatAsAtomicUnit=on
  MATLAB Function1 : MATLAB Function  TreatAsAtomicUnit=on
  Mux : Mux  Inputs=2
  Norm : Subsystem
  Terminator : Terminator
  Trigonometric Function : Trigonometry  Operator=atan2
  UTC Date Vector : Constant  Value=datevec(datetime(datetime('now', 'TimeZone','local'), 'TimeZone','Z'))  SampleTime=-1
  New Data : Outport
  Healthy : Outport  Port=2
  Fix : Outport  Port=3
  Num Satellites : Outport  Port=4
  Week : Outport  Port=5
  TOW [ms] : Outport  Port=6
  Alt WGS84 [m] : Outport  Port=7
  Alt MSL [m] : Outport  Port=8
  HDOP : Outport  Port=9
  VDOP : Outport  Port=10
  Track [rad] : Outport  Port=11
  Speed [m/s] : Outport  Port=12
  Horizontal Accuracy [m] : Outport  Port=13
  Vertical Accuracy [m] : Outport  Port=14
  Velocity Accuracy [m/s] : Outport  Port=15
  Track Accuracy [rad] : Outport  Port=16
  NED Vel [m/s] : Outport  Port=17
  Lat [rad] : Outport  Port=18
  Lon [rad] : Outport  Port=19
  wires:
  Constant/1 -> Fix/1
  Constant1/1 -> Num Satellites/1
  Constant2/1 -> Horizontal Accuracy [m]/1
  Constant3/1 -> Vertical Accuracy [m]/1
  Constant4/1 -> Velocity Accuracy [m/s]/1
  Position Noise [m]/1 -> Flat Earth to LLA/1
  Altitude WGS84 [m]/1 -> Gain/1
  Mux/1 -> Angle Conversion/1
  Angle Conversion/1 -> Flat Earth to LLA/3
  Constant5/1 -> Flat Earth to LLA/4
  "Longitude [rad] "/1 -> Mux/2
  Latitude [rad]/1 -> Mux/1
  Flat Earth to LLA/1 -> Demux2/1, Angle Conversion1/1
  Angle Conversion1/1 -> Demux/1
  Demux/2 -> Lon [rad]/1
  Demux/1 -> Lat [rad]/1
  Flat Earth to LLA/2 -> Add1/2, Alt WGS84 [m]/1
  NED Velocity [m/s]/1 -> Add2/1
  Add2/1 -> Demux3/1, NED Vel [m/s]/1
  Demux1/2 -> MATLAB Function/2(month)
  Demux1/6 -> MATLAB Function/6(second)
  UTC Date Vector/1 -> Demux1/1
  Demux1/1 -> MATLAB Function/1(year)
  Demux1/5 -> MATLAB Function/5(minute)
  Demux1/4 -> MATLAB Function/4(hour)
  Demux1/3 -> MATLAB Function/3(mday)
  MATLAB Function/2(gnss_tow) -> Gain1/1
  MATLAB Function/1(gnss_week) -> Week/1
  clock/1 -> MATLAB Function/7(sim_clock)
  Gain/1 -> Flat Earth to LLA/2
  Constant6/1 -> Healthy/1
  Trigger/1 -> New Data/1
  Gain1/1 -> TOW [ms]/1
  Demux2/1 -> Geoid Height/1
  Demux2/2 -> MATLAB Function1/1(ang)
  MATLAB Function1/1(ret) -> Geoid Height/2
  Geoid Height/1 -> Add1/1
  Add1/1 -> Alt MSL [m]/1
  Constant7/1 -> HDOP/1
  Constant8/1 -> VDOP/1
  Demux4/1 -> Trigonometric Function/2
  Demux4/2 -> Trigonometric Function/1
  Trigonometric Function/1 -> Track [rad]/1
  Velocity Noise [m/s]/1 -> Add2/2
  Constant9/1 -> Track Accuracy [rad]/1
  Demux3/1 -> Norm/1(2D Vector), Demux4/1
  Demux3/2 -> Terminator/1
  Norm/1(Norm) -> Speed [m/s]/1
